simulink model "Cartesian_MPC"  (R2018a)
settings: Solver=VariableStepAuto  StartTime=0.0  StopTime=inf  FixedStep=0.01  RelTol=1e-3  EnableMultiTasking=on
PreLoadFcn:
  | sampleTime = 0.05;
  | 
  | % Vehicle Parameters
  | R = 0.1;
  | L = 0.5;
undefined symbols (not defined in the file): C1, C2, cBW, magnitude, Waypoint
libraries: mobileRoboticsLib x2, cstblocks x1, mpclib x1, dspsrcs4 x1
settings Model: EnablePacing=on  Creator=scastro  LastModifiedBy=shravan
settings DataIOCC: LimitDataPoints=on
settings OptimizationCC: LifeSpan=inf
settings DebuggingCC: AllowSymbolicDim=off  SFUnexpectedBacktrackingDiag=warning  SFNoUnconditionalDefaultTransitionDiag=warning  SFExecutionAtInitializationDiag=none
settings CodeAppCC: StateflowObjectComments=on
settings GRTTargetCC: TargetLangStandard=C89/C90 (ANSI)  GeneratePreprocessorConditionals=Disable all
settings ConfigComp: CovMetricSettings=dw  CovHtmlReporting=on  CovSaveCumulativeToWorkspaceVar=on  CovSaveSingleToWorkspaceVar=on  CovExternalEMLEnable=off  CovSFcnEnable=off
settings SimscapeCC: SimscapeNominalValues="[{\"value\":\"10\",\"unit\":\"V\"},{\"value\":\"1\",\"unit\":\"A\"},{\"value\":\"10\",\"unit\":\"N*m\"},{\"value\":\"10\",\"unit\":\"bar\"},{\"value\":\"100\",\"unit\":\"kJ/kg\"},{\"value\":\"1\",\"unit\":\"kW\"},{\"value\":\"300\",\"unit\":\"K\"},{\"value\":\"100\",\"unit\":\"cm^3/s\"},{\"value\":\"1\",\"unit\":\"kN\"},{\"value\":\"1\",\"unit\":\"g/cm^3\"},{\"value\":\"1\",\"unit\":\"l\"},{\"value\":\"1\",\"unit\":\"cm^2\"},{\"value\":\"60\",\"unit\":\"Hz\"}]"  SimscapeLogType=all  SimscapeLogDataHistory=10000
settings ConfigurationSet: Description=SimMechanics 2G
settings ExplorerConfigSet: InternalSimMechanicsExplorerSettings="<ExplorerConfiguration><canonicalview>default</canonicalview><AnimationSetting><BasePlaybackSpeed>1.0</BasePlaybackSpeed><PlaybackSpeedFactor>1.0</PlaybackSpeedFactor></AnimationSetting><TilePanel><TileInfo><Tiles Columns=\"1\" Count=\"1\" Rows=\"1\"><Column Weight=\"1\"/><Row Weight=\"1\"/><Tile Height=\"1\" Width=\"1\" X=\"0\" Y=\"0\"/></Tiles></TileInfo><SceneInfo><SceneViewer><BGColor><R>0.60000002384185791</R><G>0.60000002384185791</G><B>0.60000002384185791</B></BGColor><Camera><DoPerspective>off</DoPerspective><Position><X>-1.70656042355848525</X><Y>-0.974920623359631922</Y><Z>4.72930454537082046</Z></Position><Center><X>0.552860638431633689</X><Y>1.42025063411503494</Y><Z>1.4843509506914252</Z></Center><Up><X>0.664249622453917166</X><Y>0.300615402055903091</Y><Z>0.684399604848363485</Z></Up><ViewLimDist>1</ViewLimDist><YLim>2.77881717169207398</YLim><XLim>3.55928742670435394</XLim></Camera></SceneViewer></SceneInfo></TilePanel><MechEditorPanel><Cameras/><GfxPanelCameraMap/><VideoCreator><PlaybackSpeedRatio>1.0</PlaybackSpeedRatio><FrameRate>30</FrameRate><VideoFormat>Motion JPEG AVI</VideoFormat><FrameSize>auto</FrameSize></VideoCreator></MechEditorPanel></ExplorerConfiguration>"

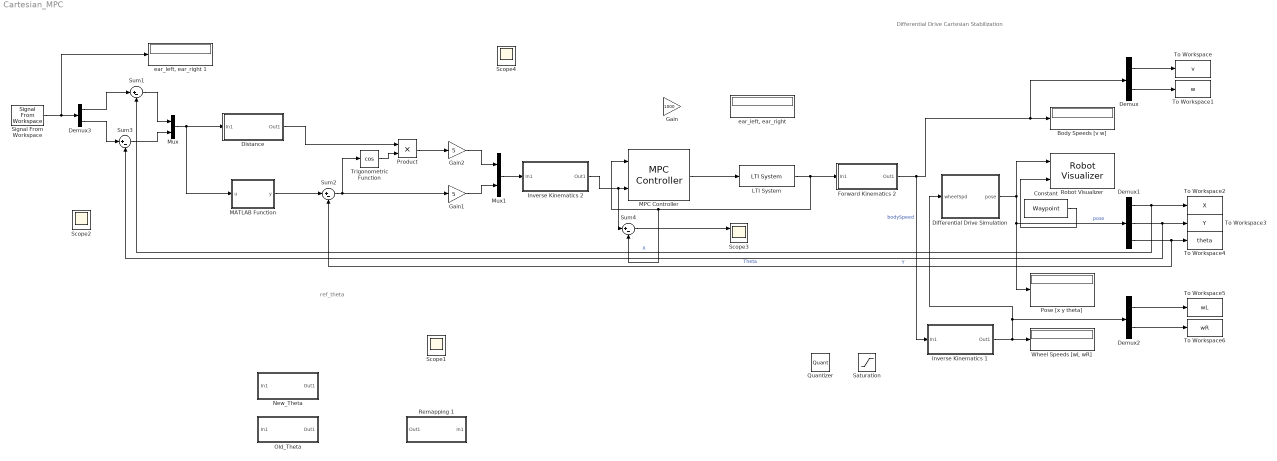
== system Cartesian_MPC ==
  note: ref_theta
  note: Differential Drive Cartesian Stabilization
  Body Speeds [v w] : Display
  Constant : Constant  Value=Waypoint  SampleTime=sampleTime
  Demux : Demux  Outputs=2
  Demux1 : Demux  Outputs=3
  Demux2 : Demux  Outputs=2
  Demux3 : Demux  Outputs=2
  Differential Drive Simulation : Subsystem  AncestorBlock=mobileRoboticsLib/Kinematic Models/Differential Drive/Differential Drive Simulation  OverrideUsingVariant=mode==2  mask(Differential Drive Simulation){wheelRadius=R, wheelBase=L, initX=C1, initY=C2, initAngle=0, Ts=sampleTime}
      mask prompts: wheelRadius "Wheel Radius [m]"; wheelBase "Wheelbase [m]"; initX "Initial X Position [m]"; initY "Initial Y Position [m]"; initAngle "Initial Angle [rad]"; Ts "Sample Time"
      mask help:
      | Simulates the kinematics of a differential drive vehicle from a specified initial pose.
      |
      | Input: Left and right wheel speeds [wL; wR], in rad/s
      |
      | Output: Pose [x; y; theta], in m, m, and rad
      |
      | Set the Sample Time parameter to 0 for continuous-time simulation, or a positive number for discrete-time simulation.
      mask Help: web('matlab:edit mrsDocDifferentialDrive')
      mask Callback Ts:
      | Ts = evalin('base',get_param(gcb,'Ts'));
      | blk = [gcb '/Generic Robot Simulation/Velocity Integrator'];
      | if Ts > 0
      |     set_param(blk,'OverrideUsingVariant','mode==2');
      | else
      |     set_param(blk,'OverrideUsingVariant','mode==1');
      | end
  "Distance " : Subsystem
  Forward Kinematics 2 : Subsystem
  Gain : Gain  Gain=1000
  Gain1 : Gain  Gain=5
  Gain2 : Gain  Gain=5
  Inverse Kinematics 1 : Subsystem
  Inverse Kinematics 2 : Subsystem
  LTI System : cstblocks/LTI System  sys=Plant  IC=[0 0 0 0]
  MATLAB Function : MATLAB Function  TreatAsAtomicUnit=on
  MPC Controller : mpclib/MPC Controller  SCDEnableBlockLinearizationSpecification=on  mpcobj=mpc1  is_multiple=0  enable_value=0  return_u0=off  updateMPCinCallerWorkspace=on  ref_from_ws=off  ref_signal_name=[]  ref_preview=off  md_from_ws=off  md_signal_name=[]  md_preview=off  from_project=off  project_file=MPCtask.mat  md_inport=off  mv_inport=off  cost_outport=off  return_sequence=off  return_qpstatus=off  return_state=off  state_inport=off  lims_inport=off  cc_inport=off  ywt_inport=off  is_designfromscratch=0  uwt_inport=off  duwt_inport=off  rhoeps_inport=off  uref_inport=off  n_ts=0.01  n_p=25  n_mv=2  n_md=0  n_ud=0  n_mo=2  n_uo=0  BlockDataType=double  SampleTimeInherited=off  switch_inport=off
  Mux : Mux  Inputs=2
  Mux1 : Mux  Inputs=2
  "New_Theta " : Subsystem
  Old_Theta : Subsystem
  Pose [x y theta] : Display
  Product : Product
  Quantizer : Quantizer
  Remapping 1 : Subsystem
  Robot Visualizer : mobileRoboticsLib/Environments/Robot Visualizer  Priority=99  robotRadius=0.8  showTrajectory=on  hasWaypoints=on  hasLidar=off  sensorOffset=[ 0 0 ]  scanAngles=[-pi/4,0,pi/4]  hasObjDetector=off  objDetectorOffset=[ 0, 0 ]  objDetectorAngle=0  objDetectorFOV=pi/4  objDetectorMaxRange=5  objectColors=[ 1, 0, 0; 0, 1, 0; 0, 0, 1 ]  objectMarkers='s'
      settings: SourceProductName=Mobile Robotics Simulation Library
  Saturation : Saturate
  Scope1 : Scope  NumInputPorts=3
  Scope2 : Scope  NumInputPorts=4
  Scope3 : Scope  NumInputPorts=2
  Scope4 : Scope  NumInputPorts=2
  Signal From Workspace : dspsrcs4/Signal From Workspace  X=Cartesian  Ts=cBW  nsamps=1  OutputAfterFinalValue=Holding final value  ignoreOrWarnInputAndFrameLengths=off  OutputFrames=off
  Sum{1..4} (4 alike) : Sum  Inputs=|+-
  To Workspace : ToWorkspace  VariableName=v  SampleTime=-1
  To Workspace1 : ToWorkspace  VariableName=w  SampleTime=-1
  To Workspace2 : ToWorkspace  VariableName=X  SampleTime=sampleTime
  To Workspace3 : ToWorkspace  VariableName=Y  SampleTime=-1
  To Workspace4 : ToWorkspace  VariableName=theta  SampleTime=-1
  To Workspace5 : ToWorkspace  VariableName=wL  SampleTime=-1
  To Workspace6 : ToWorkspace  VariableName=wR  SampleTime=-1
  Trigonometric Function : Trigonometry  Operator=cos
  Wheel Speeds [wL wR] : Display
  "ear_left, ear_right " : Display
  "ear_left, ear_right 1" : Display
  wires:
  Differential Drive Simulation/1(pose) -> Demux1/1, Pose [x y theta]/1, Robot Visualizer/1  "pose"
  Forward Kinematics 2/1(Out1) -> Inverse Kinematics 1/1(In1), Demux/1, Body Speeds [v w]/1  "bodySpeed"
  Demux/1 -> To Workspace/1
  Demux/2 -> To Workspace1/1
  Demux1/1 -> Sum1/2, To Workspace2/1  "X"
  Demux1/2 -> Sum3/2, To Workspace3/1  "Y"
  Demux2/1 -> To Workspace5/1
  Demux2/2 -> To Workspace6/1
  Gain2/1 -> Mux1/1
  Constant/1 -> Robot Visualizer/2
  Inverse Kinematics 1/1(Out1) -> Demux2/1, Differential Drive Simulation/1(wheelSpd), Wheel Speeds [wL wR]/1
  Gain1/1 -> Mux1/2
  Demux1/3 -> Sum2/2, To Workspace4/1  "Theta"
  "Distance "/1(Out1) -> Product/1
  Trigonometric Function/1 -> Product/2
  Product/1 -> Gain2/1
  Sum2/1 -> Gain1/1, Trigonometric Function/1
  Signal From Workspace/1 -> "ear_left, ear_right 1"/1, Demux3/1
  Demux3/1 -> Sum1/1
  Demux3/2 -> Sum3/1
  Sum3/1 -> Mux/2
  Sum1/1 -> Mux/1
  Mux/1 -> MATLAB Function/1(u), "Distance "/1(In1)
  Mux1/1 -> Inverse Kinematics 2/1(In1)
  LTI System/1 -> Sum4/2, MPC Controller/1, Forward Kinematics 2/1(In1)
  Inverse Kinematics 2/1(Out1) -> Sum4/1, MPC Controller/2
  MPC Controller/1 -> LTI System/1
  MATLAB Function/1(y) -> Sum2/1
  Sum4/1 -> Scope3/1

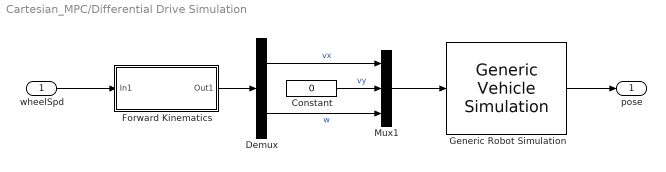
== system Cartesian_MPC/Differential Drive Simulation ==
  wheelSpd : Inport
  Constant : Constant  Value=0
  Demux : Demux  Outputs=2
  "Forward Kinematics " : Subsystem
  Generic Robot Simulation : mobileRoboticsLib/Utilities/Generic Vehicle Simulation  initX=initX  initY=initY  initAngle=initAngle  Ts=Ts
      link override Velocity Integrator: OverrideUsingVariant=mode==2
      settings: SourceProductName=Mobile Robotics Simulation Toolbox
  Mux1 : Mux  Inputs=3
  pose : Outport
  wires:
  Generic Robot Simulation/1 -> pose/1
  "Forward Kinematics "/1(Out1) -> Demux/1
  wheelSpd/1 -> "Forward Kinematics "/1(In1)
  Constant/1 -> Mux1/2  "vy"
  Demux/2 -> Mux1/3  "w"
  Demux/1 -> Mux1/1  "vx"
  Mux1/1 -> Generic Robot Simulation/1

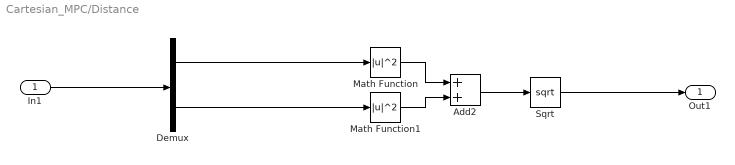
== system Cartesian_MPC/Distance  ==
  In1 : Inport
  Add2 : Sum
  Demux : Demux  Outputs=2
  Math Function : Math  Operator=magnitude^2  SaturateOnIntegerOverflow=on
  Math Function1 : Math  Operator=magnitude^2  SaturateOnIntegerOverflow=on
  Sqrt : Sqrt  SaturateOnIntegerOverflow=on
  Out1 : Outport
  wires:
  In1/1 -> Demux/1
  Demux/1 -> Math Function/1
  Demux/2 -> Math Function1/1
  Math Function/1 -> Add2/1
  Math Function1/1 -> Add2/2
  Add2/1 -> Sqrt/1
  Sqrt/1 -> Out1/1

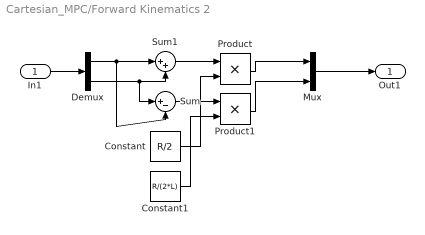
== system Cartesian_MPC/Forward Kinematics 2 ==
  In1 : Inport
  Constant : Constant  Value=R/2
  Constant1 : Constant  Value=R/(2*L)
  Demux : Demux  Outputs=2
  Mux : Mux  Inputs=2
  Product : Product
  Product1 : Product
  Sum : Sum  Inputs=|+-
  Sum1 : Sum  Inputs=|++
  Out1 : Outport
  wires:
  In1/1 -> Demux/1
  Product1/1 -> Mux/2
  Mux/1 -> Out1/1
  Product/1 -> Mux/1
  Demux/1 -> Sum/2, Sum1/1
  Demux/2 -> Sum/1, Sum1/2
  Sum1/1 -> Product/1
  Constant/1 -> Product/2
  Sum/1 -> Product1/1
  Constant1/1 -> Product1/2

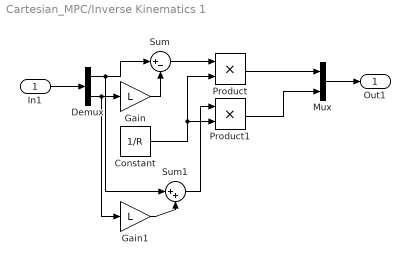
== system Cartesian_MPC/Inverse Kinematics 1 ==
  In1 : Inport
  Constant : Constant  Value=1/R
  Demux : Demux  Outputs=2
  Gain : Gain  Gain=L
  Gain1 : Gain  Gain=L
  Mux : Mux  Inputs=2
  Product : Product
  Product1 : Product
  Sum : Sum  Inputs=|+-
  Sum1 : Sum  Inputs=|++
  Out1 : Outport
  wires:
  Mux/1 -> Out1/1
  In1/1 -> Demux/1
  Demux/2 -> Gain1/1, Gain/1
  Demux/1 -> Sum1/1, Sum/1
  Gain/1 -> Sum/2
  Sum/1 -> Product/1
  Constant/1 -> Product1/2, Product/2
  Sum1/1 -> Product1/1
  Product/1 -> Mux/1
  Product1/1 -> Mux/2
  Gain1/1 -> Sum1/2

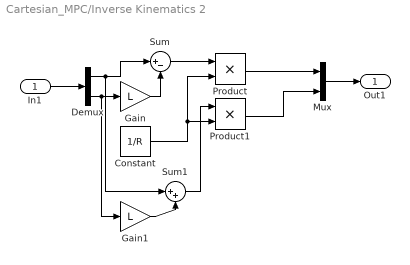
== system Cartesian_MPC/Inverse Kinematics 2 ==
  In1 : Inport
  Constant : Constant  Value=1/R
  Demux : Demux  Outputs=2
  Gain : Gain  Gain=L
  Gain1 : Gain  Gain=L
  Mux : Mux  Inputs=2
  Product : Product
  Product1 : Product
  Sum : Sum  Inputs=|+-
  Sum1 : Sum  Inputs=|++
  Out1 : Outport
  wires:
  Mux/1 -> Out1/1
  In1/1 -> Demux/1
  Demux/2 -> Gain1/1, Gain/1
  Demux/1 -> Sum1/1, Sum/1
  Gain/1 -> Sum/2
  Sum/1 -> Product/1
  Constant/1 -> Product1/2, Product/2
  Sum1/1 -> Product1/1
  Product/1 -> Mux/1
  Product1/1 -> Mux/2
  Gain1/1 -> Sum1/2

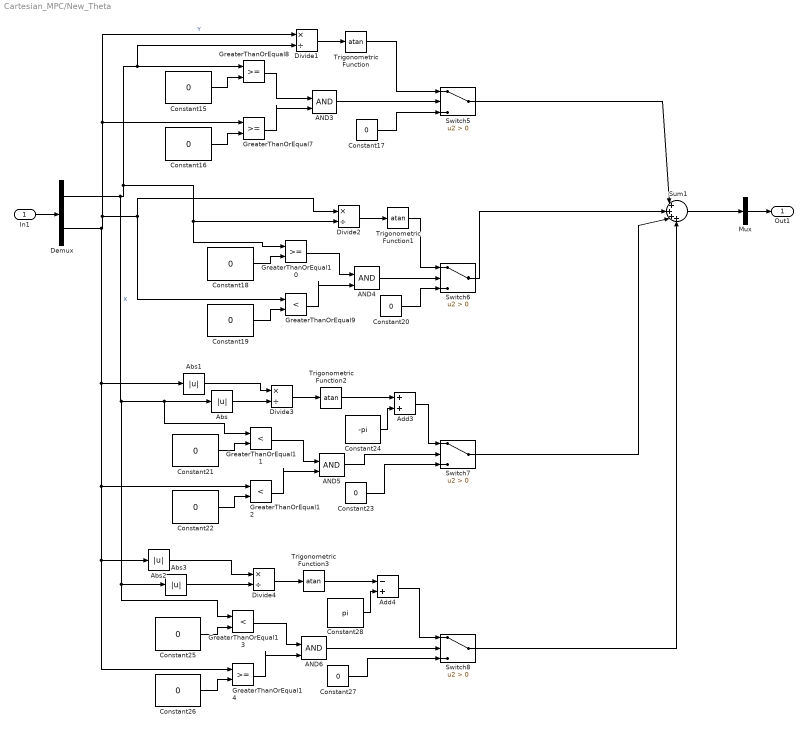
== system Cartesian_MPC/New_Theta  ==
  In1 : Inport
  AND{3..6} (4 alike) : Logic  IconShape=distinctive  AllPortsSameDT=off  OutDataTypeStr=boolean
  Abs{,1..3} (4 alike) : Abs
  Add3 : Sum
  Add4 : Sum  Inputs=-+
  Constant{15..23,25..27} (12 alike) : Constant  Value=0
  Constant24 : Constant  Value=-pi
  Constant28 : Constant  Value=pi
  Demux : Demux  Outputs=2
  Divide{1..4} (4 alike) : Product  Inputs=*/
  GreaterThanOrEqual{7..8,10,14} (4 alike) : RelationalOperator  OutDataTypeStr=boolean  RndMeth=Simplest
  GreaterThanOrEqual{9,11..13} (4 alike) : RelationalOperator  Operator=<  OutDataTypeStr=boolean  RndMeth=Simplest
  Mux : Mux  Inputs=1
  Sum1 : Sum  Inputs=|++++
  Switch{5..8} (4 alike) : Switch  Criteria=u2 > Threshold
  Trigonometric Function{,1..3} (4 alike) : Trigonometry  Operator=atan
  Out1 : Outport
  wires:
  In1/1 -> Demux/1
  Divide1/1 -> Trigonometric Function/1
  Constant16/1 -> GreaterThanOrEqual7/2
  GreaterThanOrEqual7/1 -> AND3/2
  Constant15/1 -> GreaterThanOrEqual8/2
  Demux/1 -> Abs3/1, GreaterThanOrEqual13/1, GreaterThanOrEqual11/1, Abs/1, Divide2/2, GreaterThanOrEqual10/1, Divide1/2, GreaterThanOrEqual8/1  "X"
  GreaterThanOrEqual8/1 -> AND3/1
  Constant17/1 -> Switch5/3
  AND3/1 -> Switch5/2
  Demux/2 -> GreaterThanOrEqual14/1, Abs2/1, GreaterThanOrEqual12/1, Abs1/1, GreaterThanOrEqual9/1, Divide2/1, Divide1/1, GreaterThanOrEqual7/1  "Y"
  Trigonometric Function/1 -> Switch5/1
  Trigonometric Function1/1 -> Switch6/1
  AND4/1 -> Switch6/2
  GreaterThanOrEqual10/1 -> AND4/1
  Constant19/1 -> GreaterThanOrEqual9/2
  Constant20/1 -> Switch6/3
  GreaterThanOrEqual9/1 -> AND4/2
  Constant18/1 -> GreaterThanOrEqual10/2
  Divide2/1 -> Trigonometric Function1/1
  AND5/1 -> Switch7/2
  GreaterThanOrEqual11/1 -> AND5/1
  Divide3/1 -> Trigonometric Function2/1
  GreaterThanOrEqual12/1 -> AND5/2
  Constant22/1 -> GreaterThanOrEqual12/2
  Constant21/1 -> GreaterThanOrEqual11/2
  Constant23/1 -> Switch7/3
  Trigonometric Function2/1 -> Add3/1
  Constant24/1 -> Add3/2
  Add3/1 -> Switch7/1
  Constant26/1 -> GreaterThanOrEqual14/2
  GreaterThanOrEqual14/1 -> AND6/2
  Constant28/1 -> Add4/2
  Constant27/1 -> Switch8/3
  AND6/1 -> Switch8/2
  Add4/1 -> Switch8/1
  Divide4/1 -> Trigonometric Function3/1
  GreaterThanOrEqual13/1 -> AND6/1
  Constant25/1 -> GreaterThanOrEqual13/2
  Trigonometric Function3/1 -> Add4/1
  Switch5/1 -> Sum1/1
  Switch6/1 -> Sum1/2
  Switch7/1 -> Sum1/3
  Switch8/1 -> Sum1/4
  Sum1/1 -> Mux/1
  Mux/1 -> Out1/1
  Abs1/1 -> Divide3/1
  Abs/1 -> Divide3/2
  Abs2/1 -> Divide4/1
  Abs3/1 -> Divide4/2

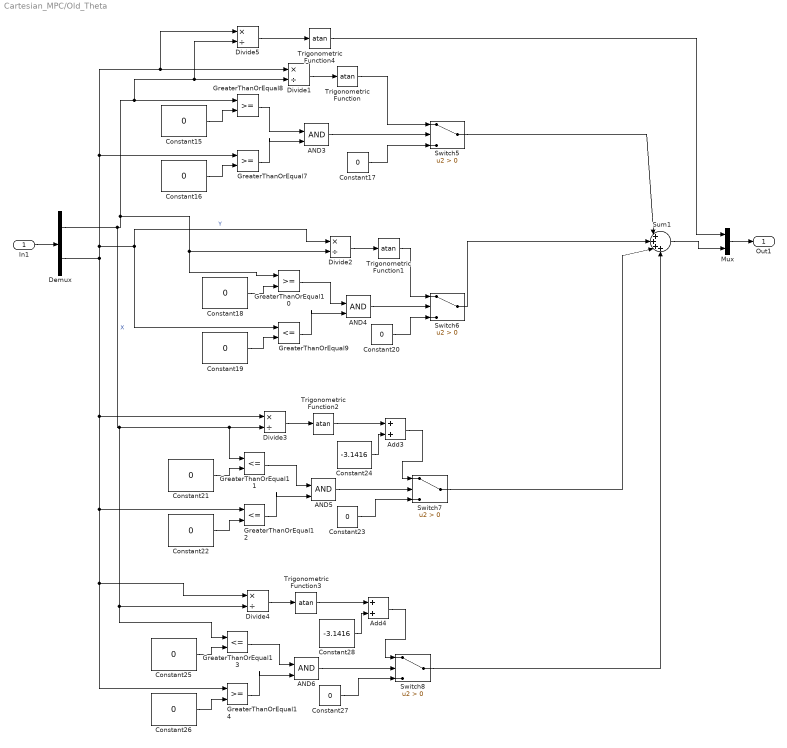
== system Cartesian_MPC/Old_Theta ==
  In1 : Inport
  AND{3..6} (4 alike) : Logic  IconShape=distinctive  AllPortsSameDT=off  OutDataTypeStr=boolean
  Add3 : Sum
  Add4 : Sum
  Constant{15..23,25..27} (12 alike) : Constant  Value=0
  Constant24 : Constant  Value=-3.1416
  Constant28 : Constant  Value=-3.1416
  Demux : Demux  Outputs=2
  Divide{1..5} (5 alike) : Product  Inputs=*/
  GreaterThanOrEqual{7..8,10,14} (4 alike) : RelationalOperator  OutDataTypeStr=boolean  RndMeth=Simplest
  GreaterThanOrEqual{9,11..13} (4 alike) : RelationalOperator  Operator=<=  OutDataTypeStr=boolean  RndMeth=Simplest
  Mux : Mux  Inputs=2
  Sum1 : Sum  Inputs=|++++
  Switch{5..8} (4 alike) : Switch  Criteria=u2 > Threshold
  Trigonometric Function{,1..4} (5 alike) : Trigonometry  Operator=atan
  Out1 : Outport
  wires:
  In1/1 -> Demux/1
  Divide1/1 -> Trigonometric Function/1
  Constant16/1 -> GreaterThanOrEqual7/2
  GreaterThanOrEqual7/1 -> AND3/2
  Constant15/1 -> GreaterThanOrEqual8/2
  Demux/1 -> Divide4/2, GreaterThanOrEqual13/1, GreaterThanOrEqual11/1, Divide3/2, Divide2/2, GreaterThanOrEqual10/1, Divide5/2, Divide1/2, GreaterThanOrEqual8/1  "X"
  GreaterThanOrEqual8/1 -> AND3/1
  Constant17/1 -> Switch5/3
  AND3/1 -> Switch5/2
  Demux/2 -> Divide4/1, GreaterThanOrEqual14/1, GreaterThanOrEqual12/1, Divide3/1, GreaterThanOrEqual9/1, Divide2/1, Divide5/1, Divide1/1, GreaterThanOrEqual7/1  "Y"
  Trigonometric Function/1 -> Switch5/1
  Trigonometric Function1/1 -> Switch6/1
  AND4/1 -> Switch6/2
  GreaterThanOrEqual10/1 -> AND4/1
  Constant19/1 -> GreaterThanOrEqual9/2
  Constant20/1 -> Switch6/3
  GreaterThanOrEqual9/1 -> AND4/2
  Constant18/1 -> GreaterThanOrEqual10/2
  Divide2/1 -> Trigonometric Function1/1
  AND5/1 -> Switch7/2
  GreaterThanOrEqual11/1 -> AND5/1
  Divide3/1 -> Trigonometric Function2/1
  GreaterThanOrEqual12/1 -> AND5/2
  Constant22/1 -> GreaterThanOrEqual12/2
  Constant21/1 -> GreaterThanOrEqual11/2
  Constant23/1 -> Switch7/3
  Trigonometric Function2/1 -> Add3/1
  Constant24/1 -> Add3/2
  Add3/1 -> Switch7/1
  Constant26/1 -> GreaterThanOrEqual14/2
  GreaterThanOrEqual14/1 -> AND6/2
  Constant28/1 -> Add4/2
  Constant27/1 -> Switch8/3
  AND6/1 -> Switch8/2
  Add4/1 -> Switch8/1
  Divide4/1 -> Trigonometric Function3/1
  GreaterThanOrEqual13/1 -> AND6/1
  Constant25/1 -> GreaterThanOrEqual13/2
  Trigonometric Function3/1 -> Add4/1
  Switch5/1 -> Sum1/1
  Switch6/1 -> Sum1/2
  Switch7/1 -> Sum1/3
  Switch8/1 -> Sum1/4
  Sum1/1 -> Mux/2
  Divide5/1 -> Trigonometric Function4/1
  Trigonometric Function4/1 -> Mux/1
  Mux/1 -> Out1/1

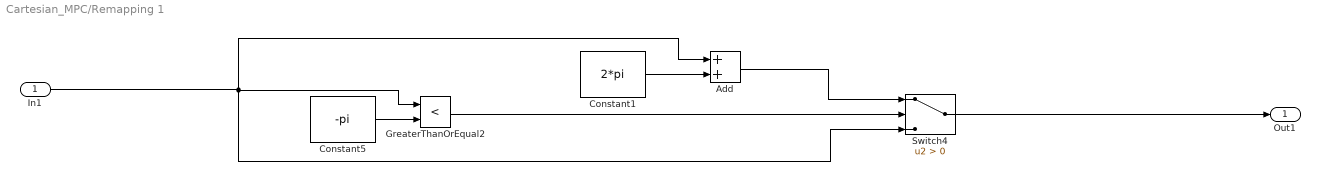
== system Cartesian_MPC/Remapping 1 ==
  In1 : Inport
  Add : Sum
  Constant1 : Constant  Value=2*pi
  Constant5 : Constant  Value=-pi
  GreaterThanOrEqual2 : RelationalOperator  Operator=<  OutDataTypeStr=boolean  RndMeth=Simplest
  Switch4 : Switch  Criteria=u2 > Threshold
  Out1 : Outport
  wires:
  In1/1 -> Switch4/3, GreaterThanOrEqual2/1, Add/1
  Constant5/1 -> GreaterThanOrEqual2/2
  Constant1/1 -> Add/2
  GreaterThanOrEqual2/1 -> Switch4/2
  Add/1 -> Switch4/1
  Switch4/1 -> Out1/1

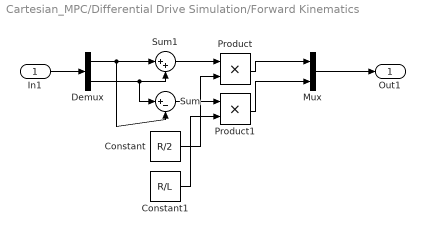
== system Cartesian_MPC/Differential Drive Simulation/Forward Kinematics  ==
  In1 : Inport
  Constant : Constant  Value=R/2
  Constant1 : Constant  Value=R/L
  Demux : Demux  Outputs=2
  Mux : Mux  Inputs=2
  Product : Product
  Product1 : Product
  Sum : Sum  Inputs=|+-
  Sum1 : Sum  Inputs=|++
  Out1 : Outport
  wires:
  In1/1 -> Demux/1
  Product1/1 -> Mux/2
  Mux/1 -> Out1/1
  Product/1 -> Mux/1
  Demux/1 -> Sum/2, Sum1/1
  Demux/2 -> Sum/1, Sum1/2
  Sum1/1 -> Product/1
  Constant/1 -> Product/2
  Sum/1 -> Product1/1
  Constant1/1 -> Product1/2

== matlab function Cartesian_MPC/MATLAB Function ==
  data: u input size=2,1; y output size=1,1
function y = fcn(u)
persistent xo yo theta;
if isempty(xo)||isempty(yo)||isempty(theta)
    xo = 1; yo = 0; theta = 0;
end
xp = u(1,1); yp = u(2,1);

% calculate the value of theta
a1 = sqrt(xp^2 + yp^2);
b1 = sqrt(xo^2 + yo^2);
c1 = sqrt((xp - xo)^2 + (yp - yo)^2);
if (a1 ~= 0)&&(b1 ~= 0)  
    dtheta = acos(max(min((a1^2 + b1^2 - c1^2)/(2*a1*b1),1),-1));
else
    dtheta = 0;
end
% calculate the direction of rotation
sign = 1;
if dtheta ~= 0
    sign = (-yo/xo)*xp + yp;
    if sign ~= 0
        if (xo > 0)&&(yo > 0)
                sign = sign/abs(sign);
        elseif (xo < 0)&&(yo < 0)
                sign = -sign/abs(sign);
        elseif (xo > 0)&&(yo < 0)
                sign = sign/abs(sign);
        elseif (xo < 0)&&(yo > 0)
                 sign = -sign/abs(sign);
        elseif (xo == 0)&&(yo >= 0)
            if xp ~= 0
                sign = -xp/abs(xp);
            else
                sign = 0;
            end
        elseif (xo == 0)&&(yo <= 0)
            if xp ~= 0
                sign = xp/abs(xp);
            else
                sign = 0;
            end
        elseif (xo >= 0)&&(yo == 0)
            if yp ~= 0
                sign = yp/abs(yp);
            else
                sign = 0;
            end
        elseif ((xo <= 0)&&(yo == 0))
            if yp ~= 0
                sign = -yp/abs(yp);
            else
                sign = 0;
            end
        end
    end
end

xo = xp; yo = yp; 
theta = theta + dtheta*sign;
y = theta;
